simulink model "cnlib"  (Simulink 6.2)
settings: Solver=ode5  SolverMode=SingleTasking  StartTime=0.0  StopTime=5  FixedStep=0.001  MaxStep=0.001  RelTol=1e-3  AbsTol=1e-3
undefined symbols (not defined in the file): k
(part 2 of 7)

== system cnlib/CN SP+Sacc +BS (5/4)/oscillating PMC ==
  note: desired
      | eye accel
  note: original parameters:
      | tau3=30ms
      | ff,fb gains = 1
  note: Robinson: PMC+ block
  note: motor
      | error
  note: efference
      | copy
  note: "Acceleration saturation" can be seen as a lookup table that
      | provides an acceleration for a given input velocity.  We then
      | use an integrator to convert the acceleration back to a velocity.
  note: From: Robinson DA, Gordon JL and Gordon SE
      | A model of smooth pursuit eye movements
      | Biological Cybernetics 55: 43-57,  1986
  note: By adding a feedback gain, and
      | matching it with a feedforward gain
      | we can make this block oscillate at
      | a lower tau3 than it would otherwise.
  desired eye vel : Inport  Port=1  LatchInput=off
  Sum : Sum  Inputs=-++  SaturateOnIntegerOverflow=on  InputSameDT=on
  Transfer Fcn2 : TransferFcn  Numerator=[3.025]  Denominator=[1 0]
  accel saturation : MATLABFcn  MATLABFcn=accsat
      mask Display: plot([-80 -4 4 80],[-120 -40 40 120], [0 0],[-120 120],[-80 80],[0 0])
  tau2 : TransportDelay  DelayTime=0.035
      mask Display: disp('35ms')
  tau3 : TransportDelay  Orientation=left  DelayTime=.040
      mask Display: disp('30ms')
  velocity noise2 : Subsystem  Orientation=up  mask(Continuous White Noise.){@1=0.0001, @2=0.001, @3=[23341]}
      mask prompts: @1 "Noise Power:"; @2 "Sample Time:"; @3 "Seed"
      mask help:
      | White noise for continuous (s-domain) systems.
      | Band-limited using zero-order-hold.
      mask init:
      | Cov = @1; Ts = @2; seed = @3; r = rand(1,12); r2 = [r(1),r;r,r(12)]; t =[1:13;1:13];
      mask Help: Implemented using white noise into Zero-Order Hold block. The seed and power can be vectors of the same length to produce a vector of white noise sources. For faster simulation, set sample time to the highest value possible but in accordance with the fastest dynamics of system.
      mask Display: plot(t(:),r2(:))
  efference copy eye vel : Outport  InitialOutput=0
  wires:
  velocity noise2/1(Out_1) -> Sum/3
  accel saturation/1 -> tau2/1
  tau2/1 -> Transfer Fcn2/1
  Sum/1 -> accel saturation/1
  tau3/1 -> Sum/1
  desired eye vel/1 -> Sum/2
  Transfer Fcn2/1 -> efference copy eye vel/1, tau3/1

== system cnlib/CN test parts/Tgt moved? ==
  PG : Inport  Port=1  LatchInput=off
  e : Inport  Port=2  LatchInput=off
  1 ms : TransportDelay  DelayTime=0.001
      mask Display: disp('1 ms')
  200 msec : TransportDelay  DelayTime=.2
      mask Display: disp('200ms')
  Derivative : Derivative
  Relational Operator1 : RelationalOperator  Operator===  InputSameDT=on
  To Workspace : ToWorkspace  VariableName=tp2  SaveFormat=Array
      settings: MaxDataPoints=10000
  To Workspace1 : ToWorkspace  VariableName=tp1  SaveFormat=Array
      settings: MaxDataPoints=10000
  To Workspace2 : ToWorkspace  VariableName=tp1a  SaveFormat=Array
      settings: MaxDataPoints=10000
  To Workspace3 : ToWorkspace  VariableName=tp2a  SaveFormat=Array
      settings: MaxDataPoints=10000
  To Workspace4 : ToWorkspace  VariableName=tp2b  SaveFormat=Array
      settings: MaxDataPoints=10000
  falling edge det : Subsystem
      mask Display: disp('Falling\nEdge Det')
  or1 : Logic
  out_1 : Outport  InitialOutput=0
  wires:
  falling edge det/1(out_1) -> 200 msec/1
  Derivative/1 -> To Workspace4/1
  e/1 -> Relational Operator1/2, Derivative/1, 1 ms/1, To Workspace/1
  Relational Operator1/1 -> or1/2, To Workspace3/1
  200 msec/1 -> or1/1, To Workspace2/1
  PG/1 -> falling edge det/1(in_1), To Workspace1/1
  or1/1 -> out_1/1
  1 ms/1 -> Relational Operator1/1

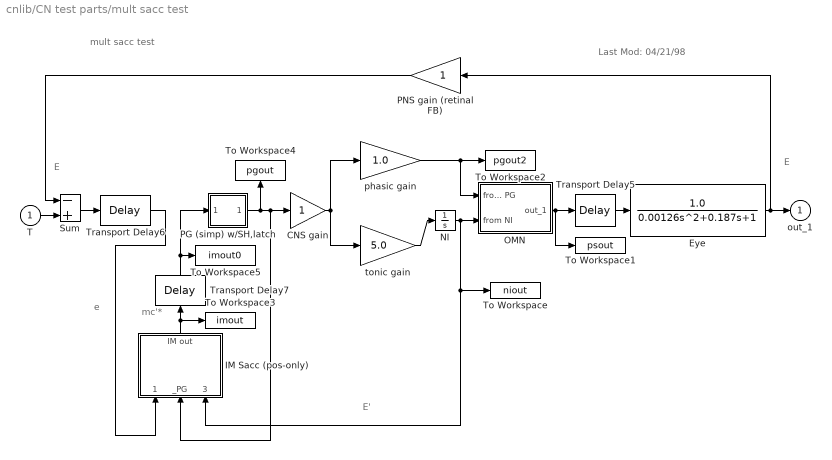
== system cnlib/CN test parts/mult sacc test ==
  note: mult sacc test
  note: mc'*
  note: E'
  note: e
  note: E
  note: E
  note: Last Mod: 04/21/98
  T : Inport  Port=1  LatchInput=off
  CNS gain : Gain  SaturateOnIntegerOverflow=on
  Eye : TransferFcn  Numerator=[1.0]  Denominator=[0.00126 0.187 1]
  IM Sacc (pos-only) : Subsystem  Orientation=up
      mask Display: disp('IM Sacc\n(pos-only)')
  NI : Integrator
  OMN : Subsystem
      mask Display: disp('<--"phasic"\nOMN\n<--"tonic"   ')
  PG (simp) w/SH,latch : Subsystem
      mask Display: disp('PG')
  PNS gain (retinal FB) : Gain  Orientation=left  SaturateOnIntegerOverflow=on
  Sum : Sum  Inputs=-+  SaturateOnIntegerOverflow=on  InputSameDT=on
  To Workspace : ToWorkspace  VariableName=niout  SaveFormat=Array
      settings: MaxDataPoints=10000
  To Workspace1 : ToWorkspace  VariableName=psout  SaveFormat=Array
      settings: MaxDataPoints=10000
  To Workspace2 : ToWorkspace  VariableName=pgout2  SaveFormat=Array
      settings: MaxDataPoints=10000
  To Workspace3 : ToWorkspace  VariableName=imout  SaveFormat=Array
      settings: MaxDataPoints=10000
  To Workspace4 : ToWorkspace  VariableName=pgout  SaveFormat=Array
      settings: Orientation=up  MaxDataPoints=10000
  To Workspace5 : ToWorkspace  VariableName=imout0  SaveFormat=Array
      settings: MaxDataPoints=10000
  Transport Delay5 : TransportDelay  DelayTime=.03
      mask Display: disp('30ms')
  Transport Delay6 : TransportDelay  DelayTime=.05
      mask Display: disp('50ms')
  Transport Delay7 : TransportDelay  Orientation=up  DelayTime=.02
      mask Display: disp('20ms')
  phasic gain : Gain  Gain=1.0  SaturateOnIntegerOverflow=on
  tonic gain : Gain  Gain=5.0  SaturateOnIntegerOverflow=on
  out_1 : Outport  InitialOutput=0
  wires:
  Sum/1 -> Transport Delay6/1
  Transport Delay5/1 -> Eye/1
  tonic gain/1 -> NI/1
  Eye/1 -> out_1/1, PNS gain (retinal FB)/1
  T/1 -> Sum/2
  PNS gain (retinal FB)/1 -> Sum/1
  OMN/1(out_1) -> Transport Delay5/1, To Workspace1/1
  CNS gain/1 -> phasic gain/1, tonic gain/1
  phasic gain/1 -> OMN/1(from PG), To Workspace2/1
  Transport Delay6/1 -> IM Sacc (pos-only)/1(_RetErr (e))
  PG (simp) w/SH,latch/1(out_1) -> CNS gain/1, IM Sacc (pos-only)/2(_PG), To Workspace4/1
  NI/1 -> OMN/2(from NI), IM Sacc (pos-only)/3(_ECPY (from NI) (E')), To Workspace/1
  IM Sacc (pos-only)/1(IM out) -> To Workspace3/1, Transport Delay7/1
  Transport Delay7/1 -> PG (simp) w/SH,latch/1(in_1), To Workspace5/1

== system cnlib/CN test parts/summing test ==
  in_1 : Inport  Port=1  LatchInput=off
  Constant : Constant  Orientation=down
  Constant2 : Constant  Orientation=up  Value=0
  Sum : Sum  SaturateOnIntegerOverflow=on  InputSameDT=on
  Switch : Switch  Threshold=.5  SaturateOnIntegerOverflow=on  InputSameDT=on
  Transport Delay : TransportDelay  Orientation=left  DelayTime=.001
  rising edge det : Subsystem
      mask Display: disp('Rising\nEdge Det')
  t : ToWorkspace  VariableName=swout  SaveFormat=Array
      mask init:
      | global t
      settings: MaxDataPoints=100000
  t1 : ToWorkspace  VariableName=detout  SaveFormat=Array
      mask init:
      | global t
      settings: MaxDataPoints=100000
  out_1 : Outport  InitialOutput=0
  wires:
  rising edge det/1(out_1) -> Switch/2, t1/1
  Switch/1 -> Sum/2, t/1
  Transport Delay/1 -> Sum/1
  Constant/1 -> Switch/1
  Constant2/1 -> Switch/3
  in_1/1 -> rising edge det/1(in_1)
  Sum/1 -> Transport Delay/1, out_1/1

== system cnlib/Harris Lib/Harris Model ==
  note: Eye Position
  note: From:  Harris, C. M. (1995). Problems in modeling congenital nystagmus: towards a new model.
      | Eye Movement Research: Mechanisms, Processes and Applications.
      | J. M. Findlay, R. Walker and R. W. Kentridge, Amsterdam, Elsevier: 239-253.
  note: Eye
      | Vel
  note: Retinal
      | Slip
      | Vel
  note: Reconstructed
      | Target
      | Velocity
  Target Velocity : Inport  Port=1  LatchInput=off
  +/-90 deg/sec : Saturate  UpperLimit=90  LowerLimit=-90
  Derivative : Derivative  Orientation=down
      mask Display: disp('s')
  Derivative1 : Derivative  Orientation=down
      mask Display: disp('s')
  Harris Plant : TransferFcn  Denominator=[.003 .262 1]
  NI : TransferFcn  Numerator=[25]  Denominator=[25 1]
  Sum : Sum  Inputs=-+  SaturateOnIntegerOverflow=on  InputSameDT=on
  Sum1 : Sum  SaturateOnIntegerOverflow=on  InputSameDT=on
  Sum2 : Sum  Orientation=up  Inputs=-+  SaturateOnIntegerOverflow=on  InputSameDT=on
  Switch : Switch  SaturateOnIntegerOverflow=on  InputSameDT=on
  a : Gain  SaturateOnIntegerOverflow=on
  b : Gain  SaturateOnIntegerOverflow=on
  c : Gain  Orientation=left  Gain=0.95  SaturateOnIntegerOverflow=on
  g : Gain  Orientation=up  SaturateOnIntegerOverflow=on
  tauc : TransportDelay  Orientation=left  DelayTime=0.050
      mask Display: disp('50ms')
  taug : TransportDelay
      mask Display: disp('80ms')
  tauv : TransportDelay  DelayTime=0.050
      mask Display: disp('50ms')
  v : Gain  SaturateOnIntegerOverflow=on
  xfer fn  1 : TransferFcn  Orientation=left  Denominator=[0.012 1]
  xfer fn  2 : TransferFcn  Orientation=up  Denominator=[0.080 1]
  Eye Pos : Outport  InitialOutput=0
  wires:
  Derivative1/1 -> xfer fn  1/1
  Target Velocity/1 -> Sum/2
  NI/1 -> Derivative1/1, b/1
  Sum1/1 -> Harris Plant/1
  a/1 -> Sum1/1
  b/1 -> Sum1/2
  Sum/1 -> tauv/1
  tauv/1 -> v/1
  v/1 -> Sum2/1
  c/1 -> Sum2/2
  tauc/1 -> c/1
  xfer fn  1/1 -> tauc/1
  Sum2/1 -> g/1
  g/1 -> xfer fn  2/1
  Derivative/1 -> Sum/1
  Harris Plant/1 -> Eye Pos/1, Derivative/1
  xfer fn  2/1 -> taug/1
  taug/1 -> +/-90 deg/sec/1
  Switch/1 -> NI/1, a/1
  +/-90 deg/sec/1 -> Switch/1

== system cnlib/Robinson CN testing/Robinson Fig. 8' ==
  note: PMC: premotor circuitry
      | CP: central processing (activity of CNS)
  note: (35ms)
  note: Robinson: Figure 8
  note: reconstructed
      | tgt vel
  note: efference
      | copy
  note: error
      | vel
  note: From: Robinson DA, Gordon JL and Gordon SE
      | A model of smooth pursuit eye movements
      | Biological Cybernetics 55: 43-57,  1986
  note: retinal feedback
  note: (loop gain = P1)
  note: "plant"
  note: (loop gain = P1 * P2)
  note: CP
  tgt vel (in) : Inport  Port=1  LatchInput=off
  P1 : Gain  Gain=.95  SaturateOnIntegerOverflow=on
  P2 : Gain  Orientation=left  SaturateOnIntegerOverflow=on
  Sum : Sum  Inputs=-++  SaturateOnIntegerOverflow=on  InputSameDT=on
  Sum1 : Sum  SaturateOnIntegerOverflow=on  InputSameDT=on
  Transfer Fcn2 : TransferFcn  Denominator=[0.07 1]
  Transfer Fcn3 : TransferFcn  Orientation=left  Denominator=[0.015 1]
  Transport Delay : TransportDelay  DelayTime=0.015
      mask Display: disp('15ms')
  Transport Delay1 : TransportDelay  DelayTime=0.03
      mask Display: disp('30ms')
  Transport Delay2 : TransportDelay  DelayTime=0.05
      mask Display: disp('50ms')
  Transport Delay3 : TransportDelay  Orientation=left  DelayTime=0.08
      mask Display: disp('80ms')
  oscillating PMC : Subsystem
      mask Display: disp('PMC')
  plant : TransferFcn  Denominator=[0.015 1]
  velocity noise : Subsystem  Orientation=up  mask(Continuous White Noise.){@1=[0.0001], @2=0.01, @3=[23341]}
      mask prompts: @1 "Noise Power:"; @2 "Sample Time:"; @3 "Seed"
      mask help:
      | White noise for continuous (s-domain) systems.
      | Band-limited using zero-order-hold.
      mask init:
      | Cov = @1; Ts = @2; seed = @3; r = rand(1,12); r2 = [r(1),r;r,r(12)]; t =[1:13;1:13];
      mask Help: Implemented using white noise into Zero-Order Hold block. The seed and power can be vectors of the same length to produce a vector of white noise sources. For faster simulation, set sample time to the highest value possible but in accordance with the fastest dynamics of system.
      mask Display: plot(t(:),r2(:))
  velocity saturation : Saturate  UpperLimit=90  LowerLimit=-90
  eye vel (out) : Outport  InitialOutput=0
  wires:
  velocity noise/1(Out_1) -> Sum/3
  Transfer Fcn2/1 -> oscillating PMC/1(desired eye vel)
  velocity saturation/1 -> Transport Delay1/1, Transfer Fcn3/1
  P1/1 -> velocity saturation/1
  oscillating PMC/1(efference copy eye vel) -> P1/1
  Transport Delay3/1 -> Sum1/1
  P2/1 -> Transport Delay3/1
  Transfer Fcn3/1 -> P2/1
  Sum/1 -> Transport Delay2/1
  Transport Delay2/1 -> Sum1/2
  Transport Delay1/1 -> plant/1
  tgt vel (in)/1 -> Sum/2
  Transport Delay/1 -> Transfer Fcn2/1
  Sum1/1 -> Transport Delay/1
  plant/1 -> Sum/1, eye vel (out)/1

== system cnlib/Robinson CN testing/original PMC ==
  note: desired
      | eye accel
  note: motor
      | error
  note: efference
      | copy
  note: Robinson: PMC block
  note: From: Robinson DA, Gordon JL and Gordon SE
      | A model of smooth pursuit eye movements
      | Biological Cybernetics 55: 43-57,  1986
  note: "Acceleration saturation" can be seen as a lookup table that
      | provides an acceleration for a given input velocity.  We then
      | use an integrator to convert the acceleration back to a velocity.
  desired eye vel : Inport  Port=1  LatchInput=off
  Sum : Sum  Inputs=-+  SaturateOnIntegerOverflow=on  InputSameDT=on
  Transfer Fcn2 : TransferFcn  Numerator=[1.1]  Denominator=[1 0]
  Transport Delay2 : TransportDelay  DelayTime=0.05
      mask Display: disp('35ms')
  Transport Delay3 : TransportDelay  Orientation=left  DelayTime=0.03
      mask Display: disp('30ms')
  accel saturation : MATLABFcn  MATLABFcn=accsat
      mask Display: plot([-80 -4 4 80],[-120 -40 40 120], [0 0],[-120 120],[-80 80],[0 0])
  efference copy eye vel : Outport  InitialOutput=0
  wires:
  accel saturation/1 -> Transport Delay2/1
  Transport Delay2/1 -> Transfer Fcn2/1
  Transfer Fcn2/1 -> efference copy eye vel/1, Transport Delay3/1
  Sum/1 -> accel saturation/1
  Transport Delay3/1 -> Sum/1
  desired eye vel/1 -> Sum/2

== system cnlib/Robinson CN testing/oscillating PMC ==
  note: By adding a feedback gain, and
      | matching it with a feedforward gain
      | we can make this block oscillate at
      | a lower tau3 than it would otherwise.
  note: From: Robinson DA, Gordon JL and Gordon SE
      | A model of smooth pursuit eye movements
      | Biological Cybernetics 55: 43-57,  1986
  note: "Acceleration saturation" can be seen as a lookup table that
      | provides an acceleration for a given input velocity.  We then
      | use an integrator to convert the acceleration back to a velocity.
  note: efference
      | copy
  note: desired
      | eye accel
  note: motor
      | error
  note: Robinson: PMC block
  note: original parameters:
      | tau3=30ms
      | ff,fb gains = 1
  desired eye vel : Inport  Port=1  LatchInput=off
  Sum : Sum  Inputs=-+  SaturateOnIntegerOverflow=on  InputSameDT=on
  Transfer Fcn2 : TransferFcn  Numerator=[1.1]  Denominator=[1 0]
  accel saturation : MATLABFcn  MATLABFcn=accsat
      mask Display: plot([-80 -4 4 80],[-120 -40 40 120], [0 0],[-120 120],[-80 80],[0 0])
  feedback : Gain  Orientation=left  SaturateOnIntegerOverflow=on
  feedfwd : Gain  SaturateOnIntegerOverflow=on
  tau2 : TransportDelay  DelayTime=0.05
      mask Display: disp('35ms')
  tau3 : TransportDelay  Orientation=left  DelayTime=.03
      mask Display: disp('30ms')
  efference copy eye vel : Outport  InitialOutput=0
  wires:
  Transfer Fcn2/1 -> feedfwd/1, feedback/1
  feedfwd/1 -> efference copy eye vel/1
  feedback/1 -> tau3/1
  desired eye vel/1 -> Sum/2
  tau3/1 -> Sum/1
  Sum/1 -> accel saturation/1
  tau2/1 -> Transfer Fcn2/1
  accel saturation/1 -> tau2/1

== system cnlib/CN IM Lib/BS Logic1/BS Enable ==
  note: BS Enable
  note: This block allows a BS for up to xx ms (set by "timer value")
      | after the acceleration criterion is met (i.e., drops below threshold)
  "ecdiff1 " : Inport  Port=1  LatchInput=off
  "[evelpr]" : Inport  Port=2  LatchInput=off
  Abs1 : Abs  SaturateOnIntegerOverflow=on
  BS Timing : Subsystem
      mask Display: disp('BS\nEnable\nTiming')
  Derivative : Derivative
      mask Display: disp('s')
  Relational Operator3 : RelationalOperator  Operator=<=  InputSameDT=on
  Switch4 : Switch  Threshold=.5  SaturateOnIntegerOverflow=on  InputSameDT=on
  To Workspace14 : ToWorkspace  VariableName=cmpr  SaveFormat=Array
      settings: MaxDataPoints=10000
      mask Type: imsw1in
  To Workspace15 : ToWorkspace  VariableName=bsenab  SaveFormat=Array
      settings: MaxDataPoints=10000
      mask Type: imsw1in
  To Workspace16 : ToWorkspace  VariableName=sout  SaveFormat=Array
      settings: MaxDataPoints=10000
      mask Type: imsw1in
  off : Constant  Orientation=up  Value=0
  threshold (accel) : Constant  Orientation=up  Value=40
  timer value : Constant  Orientation=up  Value=.035
  "[bsmc]" : Outport  InitialOutput=0
  wires:
  Relational Operator3/1 -> To Workspace14/1, BS Timing/1(From  <= [cmpr])
  Derivative/1 -> To Workspace16/1, Abs1/1
  Abs1/1 -> Relational Operator3/1
  BS Timing/1("[bsenab]") -> To Workspace15/1, Switch4/2
  "[evelpr]"/1 -> Derivative/1
  off/1 -> Switch4/3
  threshold (accel)/1 -> Relational Operator3/2
  "ecdiff1 "/1 -> Switch4/1
  Switch4/1 -> "[bsmc]"/1
  timer value/1 -> BS Timing/2(timer dur)

== system cnlib/CN IM Lib/BS Logic1/FS or BS? ==
  note: FS or BS?
  note: If the position error is _decreasing_, then the eye is approaching the
      | target, and we would like to generate a foveating saccade, since
      | this is our best time to consider capturing the target.
  note: The position error is compared to its value 5 milliseconds earlier.
      | If the error is _increasing_, we want to make a braking
      | saccade to oppose the runaway.
  pos error [ecd1str] : Inport  Port=1  LatchInput=off
  Abs : Abs  SaturateOnIntegerOverflow=on
  Relational Operator : RelationalOperator  InputSameDT=on
  Transport Delay1 : TransportDelay  DelayTime=.005
      mask Display: disp('5ms')
  BS=1 FS=0 : Outport  InitialOutput=0
  wires:
  Abs/1 -> Transport Delay1/1, Relational Operator/1
  pos error [ecd1str]/1 -> Abs/1
  Relational Operator/1 -> BS=1 FS=0/1
  Transport Delay1/1 -> Relational Operator/2

== system cnlib/CN IM Lib/BS Logic1/FS or BS?1 ==
  note: The position error is compared to its value 5 milliseconds earlier.
      | If the error is _increasing_, we want to make a braking
      | saccade to oppose the runaway.
  note: If the position error is _decreasing_, then the eye is approaching the
      | target, and we would like to generate a foveating saccade, since
      | this is our best time to consider capturing the target.
  note: FS or BS?
  pos error [ecd1str] : Inport  Port=1  LatchInput=off
  Abs : Abs  SaturateOnIntegerOverflow=on
  Relational Operator : RelationalOperator  Operator=<=  InputSameDT=on
  Transport Delay1 : TransportDelay  DelayTime=.005
      mask Display: disp('5ms')
  FS=1 BS=0 : Outport  InitialOutput=0
  wires:
  Transport Delay1/1 -> Relational Operator/2
  Relational Operator/1 -> FS=1 BS=0/1
  pos error [ecd1str]/1 -> Abs/1
  Abs/1 -> Relational Operator/1, Transport Delay1/1

== system cnlib/CN IM Lib/BS Logic1/direction ==
  in_1 : Inport  Port=1  LatchInput=off
  Constant : Constant  Value=0
  Relational Operator : RelationalOperator  Operator=>  InputSameDT=on
  Relational Operator1 : RelationalOperator  Operator=<  InputSameDT=on
  Sum : Sum  Inputs=+-  SaturateOnIntegerOverflow=on  InputSameDT=on
  out_1 : Outport  InitialOutput=0
  wires:
  Sum/1 -> out_1/1
  Relational Operator/1 -> Sum/1
  Relational Operator1/1 -> Sum/2
  Constant/1 -> Relational Operator/2, Relational Operator1/2
  in_1/1 -> Relational Operator1/1, Relational Operator/1

== system cnlib/CN IM Lib/IM (sacc) (FS+BS) (old)/FS or BS? ==
  note: The position error is compared to its value 5 milliseconds earlier.
      | If the error is _increasing_, we want to make a braking
      | saccade to oppose the runaway.
  note: If the position error is _decreasing_, then the eye is approaching the
      | target, and we would like to generate a foveating saccade, since
      | this is our best time to consider capturing the target.
  note: FS or BS?
  pos error : Inport  Port=1  LatchInput=off
  Abs : Abs  SaturateOnIntegerOverflow=on
  Relational Operator : RelationalOperator  InputSameDT=on
  Transport Delay1 : TransportDelay  DelayTime=.005
      mask Display: disp('5ms')
  FS or BS : Outport  InitialOutput=0
  wires:
  Transport Delay1/1 -> Relational Operator/2
  Relational Operator/1 -> FS or BS/1
  pos error/1 -> Abs/1
  Abs/1 -> Relational Operator/1, Transport Delay1/1

== system cnlib/CN IM Lib/IM (sacc) (FS+BS) (old) /FS or BS? ==
  note: The position error is compared to its value 5 milliseconds earlier.
      | If the error is _increasing_, we want to make a braking
      | saccade to oppose the runaway.
  note: If the position error is _decreasing_, then the eye is approaching the
      | target, and we would like to generate a foveating saccade, since
      | this is our best time to consider capturing the target.
  note: FS or BS?
  pos error : Inport  Port=1  LatchInput=off
  Abs : Abs  SaturateOnIntegerOverflow=on
  Relational Operator : RelationalOperator  Operator=<=  InputSameDT=on
  Transport Delay1 : TransportDelay  DelayTime=.005
      mask Display: disp('5ms')
  FS or BS : Outport  InitialOutput=0
  wires:
  Transport Delay1/1 -> Relational Operator/2
  Relational Operator/1 -> FS or BS/1
  pos error/1 -> Abs/1
  Abs/1 -> Relational Operator/1, Transport Delay1/1

== system cnlib/CN IM Lib/IM (sacc) (FS+BS) (old) /direction ==
  in_1 : Inport  Port=1  LatchInput=off
  Constant : Constant  Value=0
  Relational Operator : RelationalOperator  Operator=>  InputSameDT=on
  Relational Operator1 : RelationalOperator  Operator=<  InputSameDT=on
  Sum : Sum  Inputs=+-  SaturateOnIntegerOverflow=on  InputSameDT=on
  out_1 : Outport  InitialOutput=0
  wires:
  in_1/1 -> Relational Operator/1, Relational Operator1/1
  Constant/1 -> Relational Operator1/2, Relational Operator/2
  Relational Operator1/1 -> Sum/2
  Relational Operator/1 -> Sum/1
  Sum/1 -> out_1/1

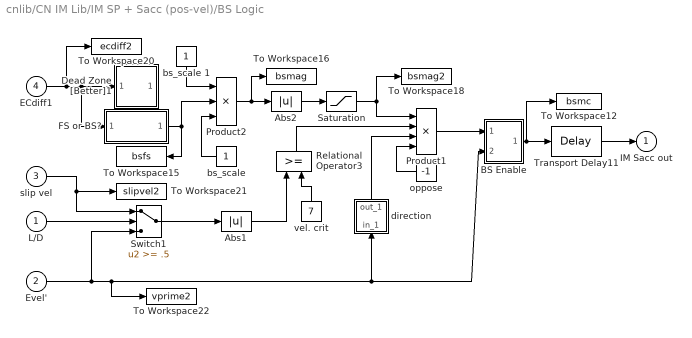
== system cnlib/CN IM Lib/IM SP + Sacc (pos-vel)/BS Logic ==
  L/D : Inport  Port=1  LatchInput=off
  Evel' : Inport  Port=2  LatchInput=off
  slip vel : Inport  Port=3  LatchInput=off
  ECdiff1 : Inport  Port=4  LatchInput=off
  Abs1 : Abs  SaturateOnIntegerOverflow=on
  Abs2 : Abs  SaturateOnIntegerOverflow=on
  BS Enable : Subsystem
      mask Display: disp('BS\nEnab')
  Dead Zone [Better]1 : Subsystem
      mask Display: disp('Dead\nZone')
  FS or BS? : Subsystem
      mask Display: disp('BS=1\nFS=0')
  Product1 : Product  Inputs=4  SaturateOnIntegerOverflow=on  RndMeth=Zero  InputSameDT=on
  Product2 : Product  Inputs=3  SaturateOnIntegerOverflow=on  RndMeth=Zero  InputSameDT=on
  Relational Operator3 : RelationalOperator  Orientation=up  InputSameDT=on
  Saturation : Saturate  UpperLimit=2  LowerLimit=0
  Switch1 : Switch  Threshold=.5  SaturateOnIntegerOverflow=on  InputSameDT=on
  To Workspace12 : ToWorkspace  VariableName=bsmc  SaveFormat=Array
      settings: MaxDataPoints=10000
  To Workspace15 : ToWorkspace  VariableName=bsfs  SaveFormat=Array
      settings: MaxDataPoints=10000
  To Workspace16 : ToWorkspace  VariableName=bsmag  SaveFormat=Array
      settings: MaxDataPoints=10000
  To Workspace18 : ToWorkspace  VariableName=bsmag2  SaveFormat=Array
      settings: MaxDataPoints=10000
  To Workspace20 : ToWorkspace  VariableName=ecdiff2  SaveFormat=Array
      settings: MaxDataPoints=10000
  To Workspace21 : ToWorkspace  VariableName=slipvel2  SaveFormat=Array
      settings: MaxDataPoints=10000
  To Workspace22 : ToWorkspace  VariableName=vprime2  SaveFormat=Array
      settings: MaxDataPoints=10000
  Transport Delay11 : TransportDelay  DelayTime=0.01
      mask Display: disp('10ms')
  "bs_scale " : Constant  Orientation=left
  bs_scale 1 : Constant  Orientation=down
  direction : Subsystem  Orientation=up
      mask Type: Sign
      mask Description: y = sign(x)
      mask Help: Sign Function:\n\t\t\ty = 1 if x > 0\n\t\t\ty = 0 if x = 0\n\t\t\ty = -1 if x < 0
      mask Display: plot(-50,-50,50,50,[-50,50],[0,0],[0,0],[-50,50],[-40,0],[-30,-30],[0,40],[30,30])
  oppose : Constant  Orientation=left  Value=-1
  vel. crit : Constant  Orientation=up  Value=7
  IM Sacc out : Outport  InitialOutput=0
  wires:
  L/D/1 -> Switch1/2
  Transport Delay11/1 -> IM Sacc out/1
  Relational Operator3/1 -> Product1/2
  Abs1/1 -> Relational Operator3/1
  vel. crit/1 -> Relational Operator3/2
  Switch1/1 -> Abs1/1
  Abs2/1 -> Saturation/1
  BS Enable/1(ecdiff (switched)) -> Transport Delay11/1, To Workspace12/1
  direction/1(out_1) -> Product1/3
  oppose/1 -> Product1/4
  Product1/1 -> BS Enable/1("ecdiff1 ")
  Saturation/1 -> To Workspace18/1, Product1/1
  Product2/1 -> To Workspace16/1, Abs2/1
  "bs_scale "/1 -> Product2/3
  FS or BS?/1(BS=1 FS=0) -> To Workspace15/1, Product2/2
  ECdiff1/1 -> FS or BS?/1(pos error), Dead Zone [Better]1/1(in_1), To Workspace20/1
  Evel'/1 -> Switch1/3, direction/1(in_1), BS Enable/2(evpr), To Workspace22/1
  slip vel/1 -> To Workspace21/1, Switch1/1
  bs_scale 1/1 -> Product2/1

== system cnlib/CN IM Lib/IM SP + Sacc (pos-vel)/Dead Zone [Better]1 ==
  note: We just output zero when the dead zone is in effect, and leave the
      |  output alone the rest of the time.
  note: This block is a better implementation of a dead zone than  the
      | block supplied by SIMULINK, because here we don't _subtract_
      | the dead zone from the rest of output.
  in_1 : Inport  Port=1  LatchInput=off
  Abs : Abs  Orientation=down  SaturateOnIntegerOverflow=on
  Relational Operator : RelationalOperator  InputSameDT=on
  Switch6 : Switch  Threshold=.5  SaturateOnIntegerOverflow=on  InputSameDT=on
  dead zone : Constant  Orientation=up
  pos (deg) criterion1 : Constant  Orientation=left  Value=0
  out_1 : Outport  InitialOutput=0
  wires:
  Relational Operator/1 -> Switch6/2
  dead zone/1 -> Relational Operator/2
  pos (deg) criterion1/1 -> Switch6/3
  Abs/1 -> Relational Operator/1
  in_1/1 -> Abs/1, Switch6/1
  Switch6/1 -> out_1/1

== system cnlib/CN IM Lib/IM SP + Sacc (pos-vel)/Dead Zone [Better]2 ==
  note: We just output zero when the dead zone is in effect, and leave the
      |  output alone the rest of the time.
  note: This block is a better implementation of a dead zone than  the
      | block supplied by SIMULINK, because here we don't _subtract_
      | the dead zone from the rest of output.
  in_1 : Inport  Port=1  LatchInput=off
  Abs : Abs  Orientation=down  SaturateOnIntegerOverflow=on
  Relational Operator : RelationalOperator  InputSameDT=on
  Switch6 : Switch  Threshold=.5  SaturateOnIntegerOverflow=on  InputSameDT=on
  dead zone : Constant  Orientation=up  Value=.2
  pos (deg) criterion1 : Constant  Orientation=left  Value=0
  out_1 : Outport  InitialOutput=0
  wires:
  Relational Operator/1 -> Switch6/2
  dead zone/1 -> Relational Operator/2
  pos (deg) criterion1/1 -> Switch6/3
  Abs/1 -> Relational Operator/1
  in_1/1 -> Abs/1, Switch6/1
  Switch6/1 -> out_1/1

== system cnlib/CN IM Lib/IM SP + Sacc (pos-vel)/ECPY enable1 ==
  note: (FF init state: Q=0)
  note: When the first PG pulse comes, its leading edge will reset the latch, and from
      | this point on, the output will be determined by the lower path
  note: If the FF init state is 0, then the block's initial output will be zero.
      | If the FF init state is 1, then the block's initial output will be one.
  _PG : Inport  Port=1  LatchInput=off
  ECPY sample : Subsystem
      mask Display: disp('ECPY\nTiming')
  Latch2 : Subsystem  mask(Latch){@1=0}
      mask prompts: @1 "Initial State for Output "Q":"
      mask help: Latch
      mask init:
      | ini=(@1~=0);
      mask Help: Latches the S input.  When S (set) is one, the Q output becomes one.  The output remains one until the R (reset) input becomes one, forcing the output to zero.  If both R and S are one, the latch will be in an undefined state.
      mask Display: disp('S   Q\n\nR  !Q')
  or : Logic  Operator=OR
  out_1 : Outport  InitialOutput=0
  wires:
  _PG/1 -> ECPY sample/1(in_1), Latch2/2(in_2)
  ECPY sample/1(out_1) -> or/2
  or/1 -> out_1/1
  Latch2/1(out_1) -> or/1

== system cnlib/CN IM Lib/IM SP + Sacc (pos-vel)/Limiter ==
  note: This block limits outputs to less than or equal to the "Limit" constant.
      | Inputs greater than "Limit" yield a zero output.
  in_1 : Inport  Port=1  LatchInput=off
  Limit : Constant  Orientation=up  Value=100
  Product : Product  SaturateOnIntegerOverflow=on  RndMeth=Zero  InputSameDT=on
  Relational Operator : RelationalOperator  Operator=<=  InputSameDT=on
  out_1 : Outport  InitialOutput=0
  wires:
  Relational Operator/1 -> Product/2
  Limit/1 -> Relational Operator/2
  Product/1 -> out_1/1
  in_1/1 -> Product/1, Relational Operator/1

== system cnlib/CN IM Lib/IM SP + Sacc (pos-vel)/OMN2 ==
  note: This block behaves like the ocular motor neurons,combining a phasic pulse (from PG)
      | with the tonic step produced by integration of the step, yielding a Pulse-Step
      | to drive the plant.
  note: Operation: when the pulse is active ("from PG") it activates the switch, passing the
      | upper input through to the output.  When the pulse is over, the switch changes,
      | allowing the lower input (from the NI) to pass.
  note: Note that the OMN properly combines the pulse with the output of the NI, by latching
      | that output to its value at the moment the pulse appears.
  note: OMN
  from NI : Inport  Port=1  LatchInput=off
  from PG : Inport  Port=2  LatchInput=off
  Abs : Abs  SaturateOnIntegerOverflow=on
  Gain _ : Gain  Gain=1.0  SaturateOnIntegerOverflow=on
  SampHold? : Subsystem
      mask Display: disp('S&H\n(L)')
  Sign : Subsystem
      mask Type: Sign
      mask Description: y = sign(x)
      mask Help: Sign Function:\n\t\t\ty = 1 if x > 0\n\t\t\ty = 0 if x = 0\n\t\t\ty = -1 if x < 0
      mask Display: plot(-50,-50,50,50,[-50,50],[0,0],[0,0],[-50,50],[-40,0],[-30,-30],[0,40],[30,30])
  Sum : Sum  SaturateOnIntegerOverflow=on  InputSameDT=on
  Switch : Switch  Threshold=.5  SaturateOnIntegerOverflow=on  InputSameDT=on
  out_1 : Outport  InitialOutput=0
  wires:
  Abs/1 -> Sign/1(in_1)
  Switch/1 -> out_1/1
  from PG/1 -> Gain _/1, Abs/1
  Sum/1 -> Switch/1
  SampHold?/1(output) -> Sum/2
  Gain _/1 -> Sum/1
  Sign/1(out_1) -> SampHold?/2(S/H?), Switch/2
  from NI/1 -> SampHold?/1(Input), Switch/3

== system cnlib/CN IM Lib/IM SP + Sacc (pos-vel)/Ret FB sample ==
  note: Retinal Feedback Sample
  note: * Output of TIMER circuit REENABLES Retinal FB
  note: * Retinal Feedback Sampling is initially ENABLED
  note: Operation:
  note: * Leading Edge of a saccade DISABLEs Retinal FB
  note: (FF init state: Q=0)
  _From PG : Inport  Port=1  LatchInput=off
  Latch1 : Subsystem  mask(Latch){@1=0}
      mask prompts: @1 "Initial State for Output "Q":"
      mask help: Latch
      mask init:
      | ini=(@1~=0);
      mask Help: Latches the S input.  When S (set) is one, the Q output  becomes one.  The output remains one until the R (reset) input becomes one, forcing the output to zero.  If both R and S are one, the latch will be in an undefined state.
      mask Display: disp('S   Q\n\nR  !Q')
  event timer2 : Subsystem
      mask Display: disp('Event\nTimer2')
  leading edge detect : Subsystem
      mask Display: disp('Leading\nEdge Det')
  timer value : Constant  Orientation=up  Value=.2
  out_1 : Outport  InitialOutput=0
  wires:
  event timer2/1(out_1) -> Latch1/2(in_2)
  leading edge detect/1(out_1) -> Latch1/1(in_1)
  Latch1/2(out_2) -> out_1/1
  _From PG/1 -> leading edge detect/1(in_1), event timer2/1(_PG)
  timer value/1 -> event timer2/2(_timer value (port))

== system cnlib/CN IM Lib/IM SP + Sacc (pos-vel)/Sacc Blank ==
  note: * Leading Edge of a saccade DISABLEs output
  note: (FF init state: Q=1)
  note: Saccade Blanking
  note: Operation:
  note: * Output is initially ENABLED
  note: * Output of TIMER circuit REENABLES output
      | ("timer value" ms after end of PG)
  _From PG : Inport  Port=1  LatchInput=off
  Latch1 : Subsystem  mask(Latch){@1=1}
      mask prompts: @1 "Initial State for Output "Q":"
      mask help: Latch
      mask init:
      | ini=(@1~=0);
      mask Help: Latches the S input.  When S (set) is one, the Q output  becomes one.  The output remains one until the R (reset) input becomes one, forcing the output to zero.  If both R and S are one, the latch will be in an undefined state.
      mask Display: disp('S   Q\n\nR  !Q')
  event timer1 : Subsystem
      mask Display: disp('Event\nTimer2')
  leading edge detect : Subsystem
      mask Display: disp('Leading\nEdge Det')
  timer value : Constant  Orientation=up  Value=.03
  out_1 : Outport  InitialOutput=0
  wires:
  timer value/1 -> event timer1/2(_timer value (port))
  Latch1/1(out_1) -> out_1/1
  _From PG/1 -> event timer1/1(_PG), leading edge detect/1(in_1)
  event timer1/1(out_1) -> Latch1/1(in_1)
  leading edge detect/1(out_1) -> Latch1/2(in_2)

== system cnlib/CN IM Lib/IM SP + Sacc (pos-vel)/SampHold? ==
  note: When "S/H?" is HIGH, then "Input" is switched directly to the
      | output ("sample").  When "S/H?" is LOW, the current output is
      | maintained ("hold").
  Input : Inport  Port=1  LatchInput=off
  S/H? : Inport  Port=2  LatchInput=off
  Memory : Memory  Orientation=left
  Sign : Subsystem
      mask Type: Sign
      mask Description: y = sign(x)
      mask Help: Sign Function:\n\t\t\ty = 1 if x > 0\n\t\t\ty = 0 if x = 0\n\t\t\ty = -1 if x < 0
      mask Display: plot(-50,-50,50,50,[-50,50],[0,0],[0,0],[-50,50],[-40,0],[-30,-30],[0,40],[30,30])
  Switch2 : Switch  Threshold=0.5  SaturateOnIntegerOverflow=on  InputSameDT=on
  output : Outport  InitialOutput=0
  wires:
  Memory/1 -> Switch2/3
  Switch2/1 -> Memory/1, output/1
  Input/1 -> Switch2/1
  Sign/1(out_1) -> Switch2/2
  S/H?/1 -> Sign/1(in_1)

== system cnlib/CN IM Lib/IM SP + Sacc (pos-vel)/SampHold?1 ==
  note: When "S/H?" is HIGH, then "Input" is switched directly to the
      | output ("sample").  When "S/H?" is LOW, the current output is
      | maintained ("hold").
  Input : Inport  Port=1  LatchInput=off
  S/H? : Inport  Port=2  LatchInput=off
  Memory : Memory  Orientation=left
  Sign : Subsystem
      mask Type: Sign
      mask Description: y = sign(x)
      mask Help: Sign Function:\n\t\t\ty = 1 if x > 0\n\t\t\ty = 0 if x = 0\n\t\t\ty = -1 if x < 0
      mask Display: plot(-50,-50,50,50,[-50,50],[0,0],[0,0],[-50,50],[-40,0],[-30,-30],[0,40],[30,30])
  Switch2 : Switch  Threshold=0.5  SaturateOnIntegerOverflow=on  InputSameDT=on
  output : Outport  InitialOutput=0
  wires:
  S/H?/1 -> Sign/1(in_1)
  Sign/1(out_1) -> Switch2/2
  Switch2/1 -> output/1, Memory/1
  Input/1 -> Switch2/1
  Memory/1 -> Switch2/3

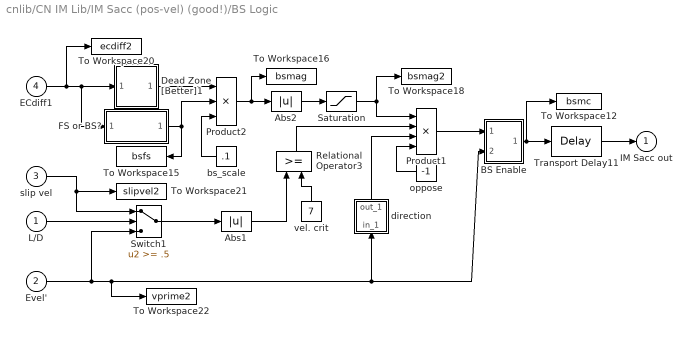
== system cnlib/CN IM Lib/IM Sacc (pos-vel) (good!)/BS Logic ==
  L/D : Inport  Port=1  LatchInput=off
  Evel' : Inport  Port=2  LatchInput=off
  slip vel : Inport  Port=3  LatchInput=off
  ECdiff1 : Inport  Port=4  LatchInput=off
  Abs1 : Abs  SaturateOnIntegerOverflow=on
  Abs2 : Abs  SaturateOnIntegerOverflow=on
  BS Enable : Subsystem
      mask Display: disp('BS\nEnab')
  Dead Zone [Better]1 : Subsystem
      mask Display: disp('Dead\nZone')
  FS or BS? : Subsystem
      mask Display: disp('BS=1\nFS=0')
  Product1 : Product  Inputs=4  SaturateOnIntegerOverflow=on  RndMeth=Zero  InputSameDT=on
  Product2 : Product  Inputs=3  SaturateOnIntegerOverflow=on  RndMeth=Zero  InputSameDT=on
  Relational Operator3 : RelationalOperator  Orientation=up  InputSameDT=on
  Saturation : Saturate  UpperLimit=2  LowerLimit=0
  Switch1 : Switch  Threshold=.5  SaturateOnIntegerOverflow=on  InputSameDT=on
  To Workspace12 : ToWorkspace  VariableName=bsmc  SaveFormat=Array
      settings: MaxDataPoints=10000
  To Workspace15 : ToWorkspace  VariableName=bsfs  SaveFormat=Array
      settings: MaxDataPoints=10000
  To Workspace16 : ToWorkspace  VariableName=bsmag  SaveFormat=Array
      settings: MaxDataPoints=10000
  To Workspace18 : ToWorkspace  VariableName=bsmag2  SaveFormat=Array
      settings: MaxDataPoints=10000
  To Workspace20 : ToWorkspace  VariableName=ecdiff2  SaveFormat=Array
      settings: MaxDataPoints=10000
  To Workspace21 : ToWorkspace  VariableName=slipvel2  SaveFormat=Array
      settings: MaxDataPoints=10000
  To Workspace22 : ToWorkspace  VariableName=vprime2  SaveFormat=Array
      settings: MaxDataPoints=10000
  Transport Delay11 : TransportDelay  DelayTime=0.01
      mask Display: disp('10ms')
  "bs_scale " : Constant  Orientation=left  Value=.1
  direction : Subsystem  Orientation=up
      mask Type: Sign
      mask Description: y = sign(x)
      mask Help: Sign Function:\n\t\t\ty = 1 if x > 0\n\t\t\ty = 0 if x = 0\n\t\t\ty = -1 if x < 0
      mask Display: plot(-50,-50,50,50,[-50,50],[0,0],[0,0],[-50,50],[-40,0],[-30,-30],[0,40],[30,30])
  oppose : Constant  Orientation=left  Value=-1
  vel. crit : Constant  Orientation=up  Value=7
  IM Sacc out : Outport  InitialOutput=0
  wires:
  L/D/1 -> Switch1/2
  Transport Delay11/1 -> IM Sacc out/1
  Relational Operator3/1 -> Product1/2
  Abs1/1 -> Relational Operator3/1
  vel. crit/1 -> Relational Operator3/2
  Switch1/1 -> Abs1/1
  Dead Zone [Better]1/1(out_1) -> Product2/1
  Abs2/1 -> Saturation/1
  direction/1(out_1) -> Product1/3
  oppose/1 -> Product1/4
  Product1/1 -> BS Enable/1("ecdiff1 ")
  BS Enable/1(ecdiff (switched)) -> Transport Delay11/1, To Workspace12/1
  Saturation/1 -> Product1/1, To Workspace18/1
  Product2/1 -> Abs2/1, To Workspace16/1
  "bs_scale "/1 -> Product2/3
  FS or BS?/1(BS=1 FS=0) -> Product2/2, To Workspace15/1
  ECdiff1/1 -> Dead Zone [Better]1/1(in_1), FS or BS?/1(pos error), To Workspace20/1
  Evel'/1 -> Switch1/3, BS Enable/2(evpr), direction/1(in_1), To Workspace22/1
  slip vel/1 -> Switch1/1, To Workspace21/1

== system cnlib/CN IM Lib/IM Sacc (pos-vel) (good!)/Dead Zone [Better] ==
  note: This block is a better implementation of a dead zone than  the
      | block supplied by SIMULINK, because here we don't _subtract_
      | the dead zone from the rest of output.
  note: We just output zero when the dead zone is in effect, and leave the
      |  output alone the rest of the time.
  in_1 : Inport  Port=1  LatchInput=off
  Abs : Abs  Orientation=down  SaturateOnIntegerOverflow=on
  Relational Operator : RelationalOperator  InputSameDT=on
  Switch6 : Switch  Threshold=.5  SaturateOnIntegerOverflow=on  InputSameDT=on
  dead zone : Constant  Orientation=up  Value=.1
  pos (deg) criterion1 : Constant  Orientation=left  Value=0
  out_1 : Outport  InitialOutput=0
  wires:
  Switch6/1 -> out_1/1
  in_1/1 -> Switch6/1, Abs/1
  Abs/1 -> Relational Operator/1
  pos (deg) criterion1/1 -> Switch6/3
  dead zone/1 -> Relational Operator/2
  Relational Operator/1 -> Switch6/2

== system cnlib/CN IM Lib/IM Sacc (pos-vel) (good!)/ECPY enable1 ==
  note: (FF init state: Q=0)
  note: When the first PG pulse comes, its leading edge will reset the latch, and from
      | this point on, the output will be determined by the lower path
  note: If the FF init state is 0, then the block's initial output will be zero.
      | If the FF init state is 1, then the block's initial output will be one.
  _PG : Inport  Port=1  LatchInput=off
  ECPY sample : Subsystem
      mask Display: disp('ECPY\nTiming')
  Latch2 : Subsystem  mask(Latch){@1=0}
      mask prompts: @1 "Initial State for Output "Q":"
      mask help: Latch
      mask init:
      | ini=(@1~=0);
      mask Help: Latches the S input.  When S (set) is one, the Q output becomes one.  The output remains one until the R (reset) input becomes one, forcing the output to zero.  If both R and S are one, the latch will be in an undefined state.
      mask Display: disp('S   Q\n\nR  !Q')
  or : Logic  Operator=OR
  out_1 : Outport  InitialOutput=0
  wires:
  _PG/1 -> Latch2/2(in_2), ECPY sample/1(in_1)
  ECPY sample/1(out_1) -> or/2
  or/1 -> out_1/1
  Latch2/1(out_1) -> or/1

== system cnlib/CN IM Lib/IM Sacc (pos-vel) (good!)/OMN2 ==
  note: This block behaves like the ocular motor neurons,combining a phasic pulse (from PG)
      | with the tonic step produced by integration of the step, yielding a Pulse-Step
      | to drive the plant.
  note: Operation: when the pulse is active ("from PG") it activates the switch, passing the
      | upper input through to the output.  When the pulse is over, the switch changes,
      | allowing the lower input (from the NI) to pass.
  note: Note that the OMN properly combines the pulse with the output of the NI, by latching
      | that output to its value at the moment the pulse appears.
  note: OMN
  from NI : Inport  Port=1  LatchInput=off
  from PG : Inport  Port=2  LatchInput=off
  Abs : Abs  SaturateOnIntegerOverflow=on
  Gain _ : Gain  Gain=1.0  SaturateOnIntegerOverflow=on
  SampHold? : Subsystem
      mask Display: disp('S&H\n(L)')
  Sign : Subsystem
      mask Type: Sign
      mask Description: y = sign(x)
      mask Help: Sign Function:\n\t\t\ty = 1 if x > 0\n\t\t\ty = 0 if x = 0\n\t\t\ty = -1 if x < 0
      mask Display: plot(-50,-50,50,50,[-50,50],[0,0],[0,0],[-50,50],[-40,0],[-30,-30],[0,40],[30,30])
  Sum : Sum  SaturateOnIntegerOverflow=on  InputSameDT=on
  Switch : Switch  Threshold=.5  SaturateOnIntegerOverflow=on  InputSameDT=on
  out_1 : Outport  InitialOutput=0
  wires:
  Abs/1 -> Sign/1(in_1)
  Switch/1 -> out_1/1
  from PG/1 -> Abs/1, Gain _/1
  Sum/1 -> Switch/1
  SampHold?/1(output) -> Sum/2
  Gain _/1 -> Sum/1
  Sign/1(out_1) -> Switch/2, SampHold?/2(S/H?)
  from NI/1 -> Switch/3, SampHold?/1(Input)

== system cnlib/CN IM Lib/IM Sacc (pos-vel) (good!)/P-V ==
  note: During PG, output velocity is zero.
  note: This block limits outputs to less than or equal to the "Limit" constant.
      | Inputs greater than "Limit" yield a zero output.
  note: Smooth Velocity
  note: This block "smooths" velocity, removing the
      | spikes associated with saccades.
  PG : Inport  Port=1  LatchInput=off
  Ret Err (vel) : Inport  Port=2  LatchInput=off
  0 : Constant  Orientation=up  Value=0
  Dead Zone [Better] : Subsystem
      mask Display: disp('Dead\nZone')
  Limiter : Subsystem
      mask Display: disp('Limiter')
  Sacc Blank : Subsystem
      mask Display: disp('Saccade\nBlanking')
  Switch : Switch  Threshold=0.5  SaturateOnIntegerOverflow=on  InputSameDT=on
  To Workspace5 : ToWorkspace  VariableName=pg15  SaveFormat=Array
      settings: Orientation=down  MaxDataPoints=10000
  To Workspace6 : ToWorkspace  VariableName=sbout  SaveFormat=Array
      settings: MaxDataPoints=10000
  To Workspace7 : ToWorkspace  VariableName=limout  SaveFormat=Array
      settings: MaxDataPoints=10000
  Transport Delay1 : TransportDelay  DelayTime=0.015
      mask Display: disp('15ms')
  v : Outport  InitialOutput=0
  wires:
  Switch/1 -> Dead Zone [Better]/1(in_1)
  Dead Zone [Better]/1(out_1) -> v/1
  Transport Delay1/1 -> Sacc Blank/1(_From PG), To Workspace5/1
  PG/1 -> Transport Delay1/1
  0/1 -> Switch/3
  Ret Err (vel)/1 -> Limiter/1(in_1)
  Limiter/1(out_1) -> To Workspace7/1, Switch/1
  Sacc Blank/1(out_1) -> Switch/2, To Workspace6/1

== system cnlib/CN IM Lib/IM Sacc (pos-vel) (good!)/Ret FB sample ==
  note: Retinal Feedback Sample
  note: * Output of TIMER circuit REENABLES Retinal FB
  note: * Retinal Feedback Sampling is initially ENABLED
  note: Operation:
  note: * Leading Edge of a saccade DISABLEs Retinal FB
  note: (FF init state: Q=0)
  _From PG : Inport  Port=1  LatchInput=off
  Latch1 : Subsystem  mask(Latch){@1=0}
      mask prompts: @1 "Initial State for Output "Q":"
      mask help: Latch
      mask init:
      | ini=(@1~=0);
      mask Help: Latches the S input.  When S (set) is one, the Q output  becomes one.  The output remains one until the R (reset) input becomes one, forcing the output to zero.  If both R and S are one, the latch will be in an undefined state.
      mask Display: disp('S   Q\n\nR  !Q')
  event timer1 : Subsystem
      mask Display: disp('Event\nTimer2')
  leading edge detect : Subsystem
      mask Display: disp('Leading\nEdge Det')
  out_1 : Outport  InitialOutput=0
  wires:
  event timer1/1(out_1) -> Latch1/2(in_2)
  leading edge detect/1(out_1) -> Latch1/1(in_1)
  Latch1/2(out_2) -> out_1/1
  _From PG/1 -> event timer1/1(_PG), leading edge detect/1(in_1)

== system cnlib/CN IM Lib/IM Sacc (pos-vel) (good!)/SampHold? ==
  note: When "S/H?" is HIGH, then "Input" is switched directly to the
      | output ("sample").  When "S/H?" is LOW, the current output is
      | maintained ("hold").
  Input : Inport  Port=1  LatchInput=off
  S/H? : Inport  Port=2  LatchInput=off
  Memory : Memory  Orientation=left
  Sign : Subsystem
      mask Type: Sign
      mask Description: y = sign(x)
      mask Help: Sign Function:\n\t\t\ty = 1 if x > 0\n\t\t\ty = 0 if x = 0\n\t\t\ty = -1 if x < 0
      mask Display: plot(-50,-50,50,50,[-50,50],[0,0],[0,0],[-50,50],[-40,0],[-30,-30],[0,40],[30,30])
  Switch2 : Switch  Threshold=0.5  SaturateOnIntegerOverflow=on  InputSameDT=on
  output : Outport  InitialOutput=0
  wires:
  Memory/1 -> Switch2/3
  Input/1 -> Switch2/1
  Switch2/1 -> Memory/1, output/1
  Sign/1(out_1) -> Switch2/2
  S/H?/1 -> Sign/1(in_1)

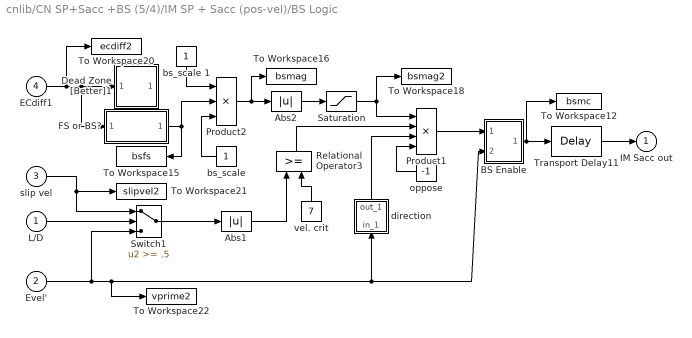
== system cnlib/CN SP+Sacc +BS (5/4)/IM SP + Sacc (pos-vel)/BS Logic ==
  L/D : Inport  Port=1  LatchInput=off
  Evel' : Inport  Port=2  LatchInput=off
  slip vel : Inport  Port=3  LatchInput=off
  ECdiff1 : Inport  Port=4  LatchInput=off
  Abs1 : Abs  SaturateOnIntegerOverflow=on
  Abs2 : Abs  SaturateOnIntegerOverflow=on
  BS Enable : Subsystem
      mask Display: disp('BS\nEnab')
  Dead Zone [Better]1 : Subsystem
      mask Display: disp('Dead\nZone')
  FS or BS? : Subsystem
      mask Display: disp('BS=1\nFS=0')
  Product1 : Product  Inputs=4  SaturateOnIntegerOverflow=on  RndMeth=Zero  InputSameDT=on
  Product2 : Product  Inputs=3  SaturateOnIntegerOverflow=on  RndMeth=Zero  InputSameDT=on
  Relational Operator3 : RelationalOperator  Orientation=up  InputSameDT=on
  Saturation : Saturate  UpperLimit=2  LowerLimit=0
  Switch1 : Switch  Threshold=.5  SaturateOnIntegerOverflow=on  InputSameDT=on
  To Workspace12 : ToWorkspace  VariableName=bsmc  SaveFormat=Array
      settings: MaxDataPoints=10000
  To Workspace15 : ToWorkspace  VariableName=bsfs  SaveFormat=Array
      settings: MaxDataPoints=10000
  To Workspace16 : ToWorkspace  VariableName=bsmag  SaveFormat=Array
      settings: MaxDataPoints=10000
  To Workspace18 : ToWorkspace  VariableName=bsmag2  SaveFormat=Array
      settings: MaxDataPoints=10000
  To Workspace20 : ToWorkspace  VariableName=ecdiff2  SaveFormat=Array
      settings: MaxDataPoints=10000
  To Workspace21 : ToWorkspace  VariableName=slipvel2  SaveFormat=Array
      settings: MaxDataPoints=10000
  To Workspace22 : ToWorkspace  VariableName=vprime2  SaveFormat=Array
      settings: MaxDataPoints=10000
  Transport Delay11 : TransportDelay  DelayTime=0.01
      mask Display: disp('10ms')
  "bs_scale " : Constant  Orientation=left
  bs_scale 1 : Constant  Orientation=down
  direction : Subsystem  Orientation=up
      mask Type: Sign
      mask Description: y = sign(x)
      mask Help: Sign Function:\n\t\t\ty = 1 if x > 0\n\t\t\ty = 0 if x = 0\n\t\t\ty = -1 if x < 0
      mask Display: plot(-50,-50,50,50,[-50,50],[0,0],[0,0],[-50,50],[-40,0],[-30,-30],[0,40],[30,30])
  oppose : Constant  Orientation=left  Value=-1
  vel. crit : Constant  Orientation=up  Value=7
  IM Sacc out : Outport  InitialOutput=0
  wires:
  bs_scale 1/1 -> Product2/1
  slip vel/1 -> Switch1/1, To Workspace21/1
  Evel'/1 -> To Workspace22/1, BS Enable/2(evpr), direction/1(in_1), Switch1/3
  ECdiff1/1 -> To Workspace20/1, Dead Zone [Better]1/1(in_1), FS or BS?/1(pos error)
  FS or BS?/1(BS=1 FS=0) -> Product2/2, To Workspace15/1
  "bs_scale "/1 -> Product2/3
  Product2/1 -> Abs2/1, To Workspace16/1
  Saturation/1 -> Product1/1, To Workspace18/1
  Product1/1 -> BS Enable/1("ecdiff1 ")
  oppose/1 -> Product1/4
  direction/1(out_1) -> Product1/3
  BS Enable/1(ecdiff (switched)) -> To Workspace12/1, Transport Delay11/1
  Abs2/1 -> Saturation/1
  Switch1/1 -> Abs1/1
  vel. crit/1 -> Relational Operator3/2
  Abs1/1 -> Relational Operator3/1
  Relational Operator3/1 -> Product1/2
  Transport Delay11/1 -> IM Sacc out/1
  L/D/1 -> Switch1/2

== system cnlib/CN SP+Sacc +BS (5/4)/IM SP + Sacc (pos-vel)/Dead Zone [Better]1 ==
  note: This block is a better implementation of a dead zone than  the
      | block supplied by SIMULINK, because here we don't _subtract_
      | the dead zone from the rest of output.
  note: We just output zero when the dead zone is in effect, and leave the
      |  output alone the rest of the time.
  in_1 : Inport  Port=1  LatchInput=off
  Abs : Abs  Orientation=down  SaturateOnIntegerOverflow=on
  Relational Operator : RelationalOperator  InputSameDT=on
  Switch6 : Switch  Threshold=.5  SaturateOnIntegerOverflow=on  InputSameDT=on
  dead zone : Constant  Orientation=up
  pos (deg) criterion1 : Constant  Orientation=left  Value=0
  out_1 : Outport  InitialOutput=0
  wires:
  Switch6/1 -> out_1/1
  in_1/1 -> Switch6/1, Abs/1
  Abs/1 -> Relational Operator/1
  pos (deg) criterion1/1 -> Switch6/3
  dead zone/1 -> Relational Operator/2
  Relational Operator/1 -> Switch6/2

== system cnlib/CN SP+Sacc +BS (5/4)/IM SP + Sacc (pos-vel)/Dead Zone [Better]2 ==
  note: This block is a better implementation of a dead zone than  the
      | block supplied by SIMULINK, because here we don't _subtract_
      | the dead zone from the rest of output.
  note: We just output zero when the dead zone is in effect, and leave the
      |  output alone the rest of the time.
  in_1 : Inport  Port=1  LatchInput=off
  Abs : Abs  Orientation=down  SaturateOnIntegerOverflow=on
  Relational Operator : RelationalOperator  InputSameDT=on
  Switch6 : Switch  Threshold=.5  SaturateOnIntegerOverflow=on  InputSameDT=on
  dead zone : Constant  Orientation=up  Value=.2
  pos (deg) criterion1 : Constant  Orientation=left  Value=0
  out_1 : Outport  InitialOutput=0
  wires:
  Switch6/1 -> out_1/1
  in_1/1 -> Switch6/1, Abs/1
  Abs/1 -> Relational Operator/1
  pos (deg) criterion1/1 -> Switch6/3
  dead zone/1 -> Relational Operator/2
  Relational Operator/1 -> Switch6/2

== system cnlib/CN SP+Sacc +BS (5/4)/IM SP + Sacc (pos-vel)/ECPY enable1 ==
  note: If the FF init state is 0, then the block's initial output will be zero.
      | If the FF init state is 1, then the block's initial output will be one.
  note: When the first PG pulse comes, its leading edge will reset the latch, and from
      | this point on, the output will be determined by the lower path
  note: (FF init state: Q=0)
  _PG : Inport  Port=1  LatchInput=off
  ECPY sample : Subsystem
      mask Display: disp('ECPY\nTiming')
  Latch2 : Subsystem  mask(Latch){@1=0}
      mask prompts: @1 "Initial State for Output "Q":"
      mask help: Latch
      mask init:
      | ini=(@1~=0);
      mask Help: Latches the S input.  When S (set) is one, the Q output becomes one.  The output remains one until the R (reset) input becomes one, forcing the output to zero.  If both R and S are one, the latch will be in an undefined state.
      mask Display: disp('S   Q\n\nR  !Q')
  or : Logic  Operator=OR
  out_1 : Outport  InitialOutput=0
  wires:
  Latch2/1(out_1) -> or/1
  or/1 -> out_1/1
  ECPY sample/1(out_1) -> or/2
  _PG/1 -> Latch2/2(in_2), ECPY sample/1(in_1)
